simulink model "Dummy"  (R2025b)
settings: Solver=VariableStepAuto  StartTime=0.0  StopTime=10.0  RelTol=1e-3
settings Model: Creator=georg  LastModifiedBy=georg

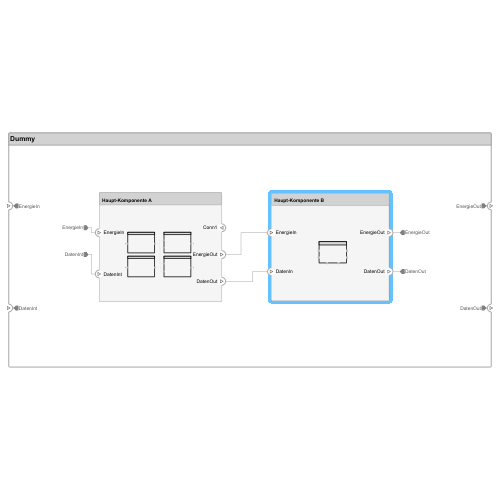
[thumbnail: Simulink's stored preview of the top-level diagram]
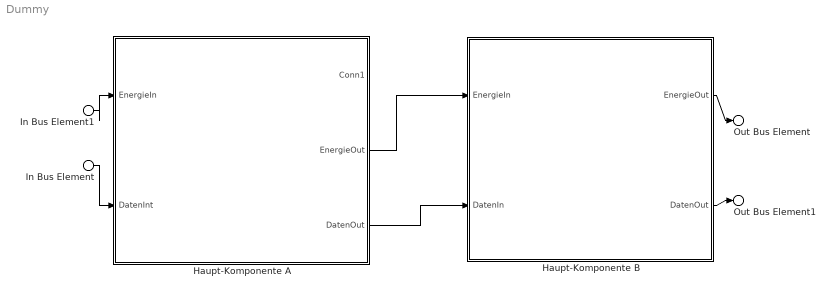
== system Dummy ==
  In Bus Element1 : Inport  PortName=EnergieIn
  In Bus Element : Inport  Port=2  PortName=DatenInt
  Haupt-Komponente A : Subsystem
      settings: PortSchema="{\"entries\":[{\"content\":{\"headerSize\":26,\"margin\":15,\"minimumSpacing\":25,\"sides\":[{\"content\":{\"connectorIds\":[\"In1\",\"In2\"]},\"type\":\"ConnectorPlacement.EquallySpacedRectSide\",\"uuid\":\"cc852fac-32eb-4011-bcf6-fcab5b2663da\"},{\"content\":{\"connectorIds\":[\"In3\",\"Out1\",\"Out2\"],\"side\":\"RIGHT\"},\"type\":\"ConnectorPlacement.EquallySpacedRectSide\",\"uuid\":\"d3171f75-c9c1-4560-973d-d39e2a90e8f6\"},{\"content\":{\"side\":\"TOP\"},\"type\":\"ConnectorPlacement.EquallySpacedRectSide\",\"uuid\":\"092262db-a7ba-48ba-a662-ee6d84045f36\"}]},\"type\":\"ConnectorPlacement.EquallySpacedConnector\",\"uuid\":\"cc59053b-a631-407b-8b33-4f9c5341cc4c\"}],\"packageUris\":[\"http://schema.mathworks.com/mf0/Connector/R2020b\"],\"version\":\"1.0\"}"
  Haupt-Komponente B : Subsystem
      settings: PortSchema="{\"entries\":[{\"content\":{\"headerSize\":26,\"margin\":15,\"minimumSpacing\":25,\"sides\":[{\"content\":{\"connectorIds\":[\"In1\",\"In2\"]},\"type\":\"ConnectorPlacement.EquallySpacedRectSide\",\"uuid\":\"cc852fac-32eb-4011-bcf6-fcab5b2663da\"},{\"content\":{\"connectorIds\":[\"Out1\",\"Out2\"],\"side\":\"RIGHT\"},\"type\":\"ConnectorPlacement.EquallySpacedRectSide\",\"uuid\":\"d3171f75-c9c1-4560-973d-d39e2a90e8f6\"},{\"content\":{\"side\":\"TOP\"},\"type\":\"ConnectorPlacement.EquallySpacedRectSide\",\"uuid\":\"092262db-a7ba-48ba-a662-ee6d84045f36\"}]},\"type\":\"ConnectorPlacement.EquallySpacedConnector\",\"uuid\":\"cc59053b-a631-407b-8b33-4f9c5341cc4c\"}],\"packageUris\":[\"http://schema.mathworks.com/mf0/Connector/R2020b\"],\"version\":\"1.0\"}"
  Out Bus Element : Outport  PortName=EnergieOut
  Out Bus Element1 : Outport  Port=2  PortName=DatenOut
  wires:
  In Bus Element1/1 -> Haupt-Komponente A/1(EnergieIn)
  Haupt-Komponente B/1(EnergieOut) -> Out Bus Element/1
  Haupt-Komponente B/2(DatenOut) -> Out Bus Element1/1
  In Bus Element/1 -> Haupt-Komponente A/2(DatenInt)
  Haupt-Komponente A/1(EnergieOut) -> Haupt-Komponente B/1(EnergieIn)
  Haupt-Komponente A/2(DatenOut) -> Haupt-Komponente B/2(DatenIn)

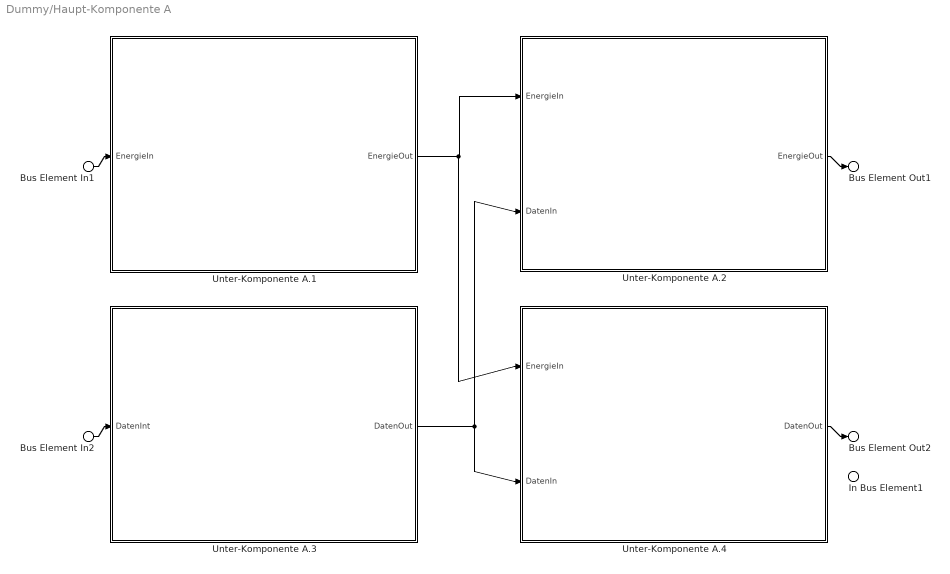
== system Dummy/Haupt-Komponente A ==
  Bus Element In1 : Inport  PortName=EnergieIn
  Bus Element In2 : Inport  Port=2  PortName=DatenInt
  In Bus Element1 : Inport  Port=3  PortName=Conn1
  Unter-Komponente A.1 : Subsystem
      settings: PortSchema="{\"entries\":[{\"content\":{\"headerSize\":26,\"margin\":15,\"minimumSpacing\":25,\"sides\":[{\"content\":{\"connectorIds\":[\"In1\"]},\"type\":\"ConnectorPlacement.EquallySpacedRectSide\",\"uuid\":\"cc852fac-32eb-4011-bcf6-fcab5b2663da\"},{\"content\":{\"connectorIds\":[\"Out1\"],\"side\":\"RIGHT\"},\"type\":\"ConnectorPlacement.EquallySpacedRectSide\",\"uuid\":\"d3171f75-c9c1-4560-973d-d39e2a90e8f6\"},{\"content\":{\"side\":\"TOP\"},\"type\":\"ConnectorPlacement.EquallySpacedRectSide\",\"uuid\":\"092262db-a7ba-48ba-a662-ee6d84045f36\"}]},\"type\":\"ConnectorPlacement.EquallySpacedConnector\",\"uuid\":\"cc59053b-a631-407b-8b33-4f9c5341cc4c\"}],\"packageUris\":[\"http://schema.mathworks.com/mf0/Connector/R2020b\"],\"version\":\"1.0\"}"
  Unter-Komponente A.2 : Subsystem
      settings: PortSchema="{\"entries\":[{\"content\":{\"headerSize\":26,\"margin\":15,\"minimumSpacing\":25,\"sides\":[{\"content\":{\"connectorIds\":[\"In1\",\"In2\"]},\"type\":\"ConnectorPlacement.EquallySpacedRectSide\",\"uuid\":\"cc852fac-32eb-4011-bcf6-fcab5b2663da\"},{\"content\":{\"connectorIds\":[\"Out1\"],\"side\":\"RIGHT\"},\"type\":\"ConnectorPlacement.EquallySpacedRectSide\",\"uuid\":\"d3171f75-c9c1-4560-973d-d39e2a90e8f6\"},{\"content\":{\"side\":\"TOP\"},\"type\":\"ConnectorPlacement.EquallySpacedRectSide\",\"uuid\":\"092262db-a7ba-48ba-a662-ee6d84045f36\"}]},\"type\":\"ConnectorPlacement.EquallySpacedConnector\",\"uuid\":\"cc59053b-a631-407b-8b33-4f9c5341cc4c\"}],\"packageUris\":[\"http://schema.mathworks.com/mf0/Connector/R2020b\"],\"version\":\"1.0\"}"
  Unter-Komponente A.3 : Subsystem
      settings: PortSchema="{\"entries\":[{\"content\":{\"headerSize\":26,\"margin\":15,\"minimumSpacing\":25,\"sides\":[{\"content\":{\"connectorIds\":[\"In1\"]},\"type\":\"ConnectorPlacement.EquallySpacedRectSide\",\"uuid\":\"cc852fac-32eb-4011-bcf6-fcab5b2663da\"},{\"content\":{\"connectorIds\":[\"Out1\"],\"side\":\"RIGHT\"},\"type\":\"ConnectorPlacement.EquallySpacedRectSide\",\"uuid\":\"d3171f75-c9c1-4560-973d-d39e2a90e8f6\"},{\"content\":{\"side\":\"TOP\"},\"type\":\"ConnectorPlacement.EquallySpacedRectSide\",\"uuid\":\"092262db-a7ba-48ba-a662-ee6d84045f36\"}]},\"type\":\"ConnectorPlacement.EquallySpacedConnector\",\"uuid\":\"cc59053b-a631-407b-8b33-4f9c5341cc4c\"}],\"packageUris\":[\"http://schema.mathworks.com/mf0/Connector/R2020b\"],\"version\":\"1.0\"}"
  Unter-Komponente A.4 : Subsystem
      settings: PortSchema="{\"entries\":[{\"content\":{\"headerSize\":26,\"margin\":15,\"minimumSpacing\":25,\"sides\":[{\"content\":{\"connectorIds\":[\"In1\",\"In2\"]},\"type\":\"ConnectorPlacement.EquallySpacedRectSide\",\"uuid\":\"cc852fac-32eb-4011-bcf6-fcab5b2663da\"},{\"content\":{\"connectorIds\":[\"Out1\"],\"side\":\"RIGHT\"},\"type\":\"ConnectorPlacement.EquallySpacedRectSide\",\"uuid\":\"d3171f75-c9c1-4560-973d-d39e2a90e8f6\"},{\"content\":{\"side\":\"TOP\"},\"type\":\"ConnectorPlacement.EquallySpacedRectSide\",\"uuid\":\"092262db-a7ba-48ba-a662-ee6d84045f36\"}]},\"type\":\"ConnectorPlacement.EquallySpacedConnector\",\"uuid\":\"cc59053b-a631-407b-8b33-4f9c5341cc4c\"}],\"packageUris\":[\"http://schema.mathworks.com/mf0/Connector/R2020b\"],\"version\":\"1.0\"}"
  Bus Element Out1 : Outport  PortName=EnergieOut
  Bus Element Out2 : Outport  Port=2  PortName=DatenOut
  wires:
  Bus Element In1/1 -> Unter-Komponente A.1/1(EnergieIn)
  Bus Element In2/1 -> Unter-Komponente A.3/1(DatenInt)
  Unter-Komponente A.2/1(EnergieOut) -> Bus Element Out1/1
  Unter-Komponente A.4/1(DatenOut) -> Bus Element Out2/1
  Unter-Komponente A.1/1(EnergieOut) -> Unter-Komponente A.4/1(EnergieIn), Unter-Komponente A.2/1(EnergieIn)
  Unter-Komponente A.3/1(DatenOut) -> Unter-Komponente A.2/2(DatenIn), Unter-Komponente A.4/2(DatenIn)

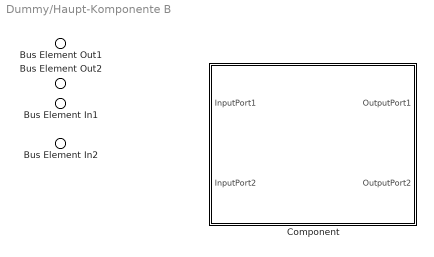
== system Dummy/Haupt-Komponente B ==
  Bus Element In1 : Inport  PortName=EnergieIn
  Bus Element In2 : Inport  Port=2  PortName=DatenIn
  Component : Subsystem
      settings: PortSchema="{\"entries\":[{\"content\":{\"headerSize\":26,\"margin\":15,\"minimumSpacing\":25,\"sides\":[{\"content\":{\"connectorIds\":[\"In1\",\"In2\"]},\"type\":\"ConnectorPlacement.EquallySpacedRectSide\",\"uuid\":\"8d645fa3-2e17-47d6-b57c-061bf9ca2ad7\"},{\"content\":{\"connectorIds\":[\"Out1\",\"Out2\"],\"side\":\"RIGHT\"},\"type\":\"ConnectorPlacement.EquallySpacedRectSide\",\"uuid\":\"da1024a9-13df-487c-8b1b-4ef52eaa82ca\"},{\"content\":{\"side\":\"TOP\"},\"type\":\"ConnectorPlacement.EquallySpacedRectSide\",\"uuid\":\"4b7ed5f6-e467-4f05-b247-196e9d305cb8\"},{\"content\":{\"connectorIds\":[\"RConn1\",\"RConn2\"],\"side\":\"BOTTOM\"},\"type\":\"ConnectorPlacement.EquallySpacedRectSide\",\"uuid\":\"e5db2f2a-c3b1-468f-ab30-6f677bcb4929\"}]},\"type\":\"ConnectorPlacement.EquallySpacedConnector\",\"uuid\":\"d256ca4d-3894-42a0-b30b-ffcbc62b7626\"}],\"packageUris\":[\"http://schema.mathworks.com/mf0/Connector/R2020b\"],\"version\":\"1.0\"}"
  Bus Element Out1 : Outport  PortName=EnergieOut
  Bus Element Out2 : Outport  Port=2  PortName=DatenOut

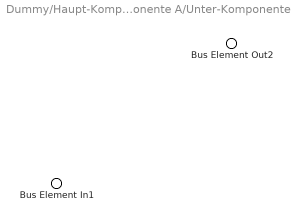
== system Dummy/Haupt-Komponente A/Unter-Komponente A.1 ==
  Bus Element In1 : Inport  PortName=EnergieIn
  Bus Element Out2 : Outport  PortName=EnergieOut

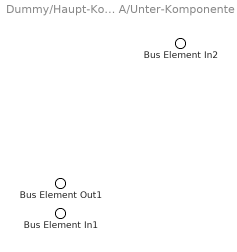
== system Dummy/Haupt-Komponente A/Unter-Komponente A.2 ==
  Bus Element In2 : Inport  PortName=EnergieIn
  Bus Element In1 : Inport  Port=2  PortName=DatenIn
  Bus Element Out1 : Outport  PortName=EnergieOut

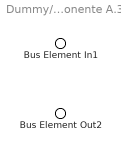
== system Dummy/Haupt-Komponente A/Unter-Komponente A.3 ==
  Bus Element In1 : Inport  PortName=DatenInt
  Bus Element Out2 : Outport  PortName=DatenOut

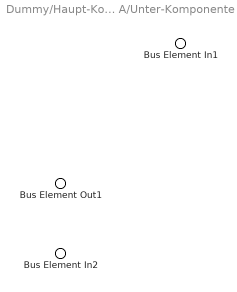
== system Dummy/Haupt-Komponente A/Unter-Komponente A.4 ==
  Bus Element In1 : Inport  PortName=EnergieIn
  Bus Element In2 : Inport  Port=2  PortName=DatenIn
  Bus Element Out1 : Outport  PortName=DatenOut

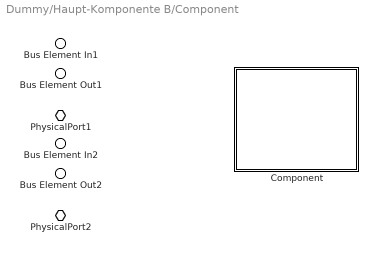
== system Dummy/Haupt-Komponente B/Component ==
  Bus Element In1 : Inport  PortName=InputPort1
  Bus Element In2 : Inport  Port=2  PortName=InputPort2
  Component : Subsystem
      settings: PortSchema="{\"entries\":[{\"content\":{\"headerSize\":26,\"margin\":15,\"minimumSpacing\":25,\"sides\":[{\"content\":{},\"type\":\"ConnectorPlacement.EquallySpacedRectSide\",\"uuid\":\"8d645fa3-2e17-47d6-b57c-061bf9ca2ad7\"},{\"content\":{\"side\":\"RIGHT\"},\"type\":\"ConnectorPlacement.EquallySpacedRectSide\",\"uuid\":\"da1024a9-13df-487c-8b1b-4ef52eaa82ca\"},{\"content\":{\"side\":\"TOP\"},\"type\":\"ConnectorPlacement.EquallySpacedRectSide\",\"uuid\":\"4b7ed5f6-e467-4f05-b247-196e9d305cb8\"}]},\"type\":\"ConnectorPlacement.EquallySpacedConnector\",\"uuid\":\"d256ca4d-3894-42a0-b30b-ffcbc62b7626\"}],\"packageUris\":[\"http://schema.mathworks.com/mf0/Connector/R2020b\"],\"version\":\"1.0\"}"
  PhysicalPort1 : PMIOPort  Side=Right
  PhysicalPort2 : PMIOPort  Port=2  Side=Right
  Bus Element Out1 : Outport  PortName=OutputPort1
  Bus Element Out2 : Outport  Port=2  PortName=OutputPort2

== system Dummy/Haupt-Komponente B/Component/Component ==
